simulink model "mconversion4"  (Simulink 8.0)
settings: Solver=FixedStepDiscrete  StartTime=0.0  StopTime=10.0  RelTol=1e-3
libraries: mconversion4Lib x2
settings Model: Creator=awarlock  LastModifiedBy=htu  ExtModeAutoUpdateStatusClock=off
settings DataIOCC: SignalLoggingSaveFormat=ModelDataLogs  SignalLoggingName=logsOut
settings OptimizationCC: InlineParams=on  InlineInvariantSignals=on  InitFltsAndDblsToZero=on  OptimizeModelRefInitCode=on  LifeSpan=1
settings DebuggingCC: SaveWithParameterizedLinksMsg=none  CheckExecutionContextPreStartOutputMsg=on  CheckExecutionContextRuntimeOutputMsg=on  SignalResolutionControl=TryResolveAllWithWarning  SolverPrmCheckMsg=none  MultiTaskDSMMsg=warning  MultiTaskCondExecSysMsg=none
settings HardwareCC: ProdHWDeviceType=Specified  TargetHWDeviceType=32-bit Generic  ProdEqTarget=off
settings RTWCC: SystemTargetFile=ert.tlc  TemplateMakefile=ert_default_tmf  Description=RTW Embedded Coder (no auto configuration)  ProcessScript=ert_make_rtw_hook  IncludeERTFirstTime=on
settings CodeAppCC: IgnoreCustomStorageClasses=off
settings ERTTargetCC: TargetFcnLib=ansi_tfl_tmw.mat  CodeReplacementLibrary=ANSI_C  MultiwordLength=2048  GenerateSampleERTMain=on  SupportContinuousTime=on  SupportNonInlinedSFcns=on  ERTCustomFileTemplate=example_file_process.tlc  ConvertIfToSwitch=off  SuppressUnreachableDefaultCases=off

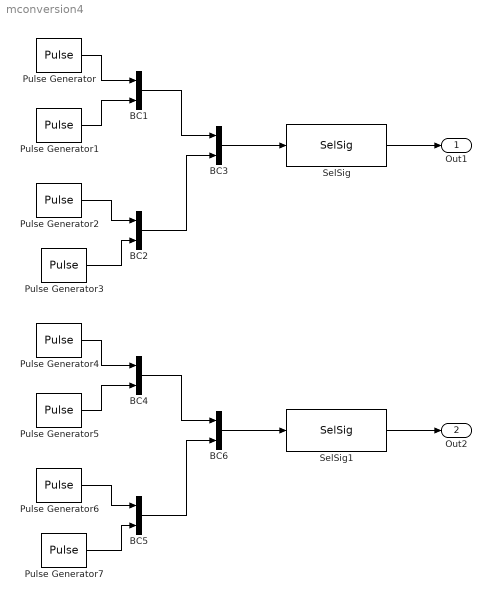
== system mconversion4 ==
  BC{1..6} (6 alike) : BusCreator  DialogController=Simulink.DDGSource_Bus  Inputs=2
  Pulse Generator : DiscretePulseGenerator
  Pulse Generator1 : DiscretePulseGenerator  Amplitude=2
  Pulse Generator2 : DiscretePulseGenerator  Amplitude=3
  Pulse Generator3 : DiscretePulseGenerator  Amplitude=4
  Pulse Generator4 : DiscretePulseGenerator  Amplitude=5
  Pulse Generator5 : DiscretePulseGenerator  Amplitude=6
  Pulse Generator6 : DiscretePulseGenerator  Amplitude=7
  Pulse Generator7 : DiscretePulseGenerator  Amplitude=8
  SelSig : mconversion4Lib/SelSig
  SelSig1 : mconversion4Lib/SelSig
  Out1 : Outport
  Out2 : Outport  Port=2
  wires:
  Pulse Generator/1 -> BC1/1
  Pulse Generator1/1 -> BC1/2
  Pulse Generator2/1 -> BC2/1
  Pulse Generator3/1 -> BC2/2
  BC1/1 -> BC3/1
  BC2/1 -> BC3/2
  BC3/1 -> SelSig/1
  SelSig/1 -> Out1/1
  Pulse Generator4/1 -> BC4/1
  Pulse Generator5/1 -> BC4/2
  Pulse Generator6/1 -> BC5/1
  Pulse Generator7/1 -> BC5/2
  BC4/1 -> BC6/1
  BC5/1 -> BC6/2
  BC6/1 -> SelSig1/1
  SelSig1/1 -> Out2/1
